simulink model "QD2_DroneStack_PID_2021a"  (R2026a)
settings: Solver=ode1  StopTime=inf  FixedStep=1/1000  EnableMultiTasking=on
InitFcn:
  | Motor_Mapping_7_Inch
model workspace (MAT data in the model file):
  target_system = 1
undefined symbols (not defined in the file): _Commander, _Stabilizer, _SYSID, datetime, HIL, KT, lf, log_, log_QD2_, m, Motor_Matrix, n, qc_get_step_size, s, saved_data
libraries: quarc_library x107, simulink x30, simulink_extras x3, sl_discontinuities x2
(part 5 of 5)

== matlab function QD2_DroneStack_PID_2021a/COMMANDER (ANGLE MODE)/STATE MACHINE TRANSITION ==
  data: current_state input; E_Abort input; isArm input; pt_ARM_to_TAKEOFF_THROTTLE input; pt_TAKE_OFF_HEIGHT_TO_AUTOLAND input; pt_FLIGHT_TO_AUTOLAND input; Next_state output; pt_TAKEOFF_THROTTLE_TO_TAKEOFF_HEIGHT input; pt_TAKE_OFF_HEIGHT_TO_FLIGHT input; pt_AUTOLAND_TO_DISABLE input; pt_EMERGENCY_STOP_TO_DISABLE input; pt_EMERGENCY_ABORT_TO_DISABLE input; Error input
function Next_state = SM_transition(current_state, E_Abort, isArm, pt_ARM_to_TAKEOFF_THROTTLE, pt_TAKE_OFF_HEIGHT_TO_AUTOLAND, pt_FLIGHT_TO_AUTOLAND, pt_TAKEOFF_THROTTLE_TO_TAKEOFF_HEIGHT, pt_TAKE_OFF_HEIGHT_TO_FLIGHT, pt_AUTOLAND_TO_DISABLE, pt_EMERGENCY_STOP_TO_DISABLE, pt_EMERGENCY_ABORT_TO_DISABLE, Error)

% Programmatic Transition Block
%
% FINITE STATE MACHINE (FSM) with 9 states as described below, transitioning based on the 
% values of the isArm, transition signals, Error, and E_Abort
%
% Last modified: March, 2020
%
% INPUTS:
% ------
% current_state = Current state of the FSM        (#)     [1]
% E_Abort                                         (bool)  [1]
% isArm                                           (bool)  [1]
% pt_ARM_TO_TAKEOFF_THROTTLE                      (bool)  [1]
% pt_TAKE_OFF_HEIGHT_TO_AUTOLAND                  (bool)  [1]
% pt_FLIGHT_TO_AUTOLAND                           (bool)  [1]
% pt_TAKEOFF_THROTTLE_TO_TAKEOFF_HEIGHT           (bool)  [1]
% pt_TAKE_OFF_HEIGHT_TO_FLIGHT                    (bool)  [1]
% pt_AUTOLAND_TO_DISABLE                          (bool)  [1]
% pt_EMERGENCY_STOP_TO_DISABLE                    (bool)  [1]
% pt_EMERGENCY_ABORT_TO_DISABLE                   (bool)  [1]
% Error                                           (bool)  [1]
%
% OUTPUT:
% -------
% Next_state = Next state of the FSM              (#)     [1]

Next_state = double(0);
switch current_state
%-------------------------------------------------------------------------%
    case 1 % IDLE STATE
        if E_Abort
            Next_state = 8; % GOTO EMERGENCY ABORT STATE
        elseif Error
            Next_state = 7; % GOTO EMERGENCY STOP STATE
        elseif isArm
            Next_state = 2; % GOTO ARMED STATE
        else
            Next_state = 1; % STAY IN IDLE STATE
        end
%-------------------------------------------------------------------------%
    case 2 % ARMED STATE
        if E_Abort
            Next_state = 8; % GOTO EMERGENCY ABORT STATE
        elseif Error
            Next_state = 7; % GOTO EMERGENCY STOP STATE
        elseif ~isArm
            Next_state = 1; % GOTO IDLE STATE
        elseif pt_ARM_to_TAKEOFF_THROTTLE
            Next_state = 3; % GOTO TAKEOFF_THROTTLE STATE 
        else
            Next_state = 2; % STAY IN ARMED STATE
        end
%-------------------------------------------------------------------------%
    case 3 % TAKEOFF_THROTTLE STATE
        if E_Abort
            Next_state = 8; % GOTO EMERGENCY ABORT STATE
        elseif Error
            Next_state = 7; % GOTO EMERGENCY STOP STATE
        elseif pt_TAKEOFF_THROTTLE_TO_TAKEOFF_HEIGHT
            Next_state = 4; % GOTO TAKEOFF_HEIGHT STATE
        else
            Next_state = 3; % STAY IN TAKEOFF_THROTTLE STATE
        end
%-------------------------------------------------------------------------%
    case 4 % TAKEOFF_HEIGHT STATE
        if E_Abort
            Next_state = 8; % GOTO EMERGENCY ABORT STATE
        elseif Error
            Next_state = 7; % GOTO EMERGENCY STOP STATE
        elseif pt_TAKE_OFF_HEIGHT_TO_AUTOLAND
            Next_state = 6;
        elseif pt_TAKE_OFF_HEIGHT_TO_FLIGHT
            Next_state = 5; % GOTO FLIGHT STATE
        else
            Next_state = 4; % STAY IN TAKEOFF_HEIGHT STATE
        end
%-------------------------------------------------------------------------%
    case 5 % FLIGHT STATE
        if E_Abort
            Next_state = 8; % GOTO EMERGENCY ABORT STATE
        elseif Error
            Next_state = 7; % GOTO EMERGENCY STOP STATE
        elseif pt_FLIGHT_TO_AUTOLAND
            Next_state = 6; % GOTO AUTO_LAND STATE
        else
            Next_state = 5; % STAY IN FLIGHT STATE
        end
%-------------------------------------------------------------------------%       
    case 6 % AUTO_LAND STATE
        if E_Abort
            Next_state = 8; % GOTO EMERGENCY ABORT STATE
        elseif Error
            Next_state = 7; % GOTO EMERGENCY STOP STATE
        elseif pt_AUTOLAND_TO_DISABLE
            Next_state = 9; % GOTO DISABLE STATE
        else
            Next_state = 6; % STAY IN AUTO_LAND STATE
        end
%-------------------------------------------------------------------------%
    case 7 % EMERGENCY STOP STATE
        if E_Abort
            Next_state = 8; % GOTO EMERGENCY ABORT STATE
        elseif pt_EMERGENCY_STOP_TO_DISABLE
            Next_state = 9; % GOTO DISABLE STATE
        else
            Next_state = 7; % STAY IN EMERGENCY STOP STATE
        end
%-------------------------------------------------------------------------%
    case 8 % EMERGENCY ABORT
        if pt_EMERGENCY_ABORT_TO_DISABLE
            Next_state = 9; % GOTO DISABLE STATE
        else 
            Next_state = 8; % STAY IN EMERGENCY ABORT STATE
        end
%-------------------------------------------------------------------------%    
    case 9 % DISABLE
        Next_state = 9; % Always stay in DISABLE state if you are here    
end

== matlab function QD2_DroneStack_PID_2021a/Communication/Detect Communication Loss/MATLAB Function ==
  settings: updateMethod=DISCRETE
  data: time input; stream_connection_loss output; state input; error input; ms_time input; data_loss output
function [stream_connection_loss , data_loss] = fcn(time, state, error, ms_time)

persistent ms_time_prev
    if isempty(ms_time_prev)
        ms_time_prev = 0;
    end

stream_connection_loss = 0;
data_loss = 0;
if time > 3
    if ((state ~= 2)&&(error < 0))
        % stream connection is not established correctly
        stream_connection_loss = 1;
    end

    if (ms_time == ms_time_prev)&&(ms_time > 0)
        % data is stale
        data_loss = 1;
    end
end

ms_time_prev = ms_time;

== matlab function QD2_DroneStack_PID_2021a/QDrone 2 DAQ/Attitude Estimate from IMU Data/For Each Subsystem - Iterate over IMU0 and IMU1/Roll and Pitch Approximation from Accelerometer data ==
  data: acc_body input; roll_acc output; pitch_acc output
function [roll_acc, pitch_acc]   = fcn(acc_body)
%#eml
n = norm(acc_body,2);
if n>eps
    acc_body = acc_body/n; 
else
    acc_body = [0 0 1]';
end

roll_acc = atan2(acc_body(2),acc_body(3));
pitch_acc = atan2( -acc_body(1), acc_body(2)*sin(roll_acc)+acc_body(3)*cos(roll_acc));

== matlab function QD2_DroneStack_PID_2021a/QDrone 2 DAQ/Choose Motor Telemetry/MATLAB Function ==
  data: enable input; idx output; n input
function idx = num_seq(enable, n)

% Generate a running sequence of number from 0 to n
persistent state 

if isempty(state)
    state = 0;
end

% Output state index
idx = state;

if enable
    % Increment state index
    state = state + 1;
    % Check state index, reset when needed
    if state >= n
        state = 0;
    end
else
    % reset state to zero and not requesting telemetry
    state = 0;
    idx = 0;
end

== matlab function QD2_DroneStack_PID_2021a/QDrone 2 DAQ/Detect ESC Problems/MATLAB Function ==
  settings: updateMethod=DISCRETE  sampleTime=qc_get_step_size
  data: u input; n output; buffer_size input
function n = count_pulses(u, buffer_size)

persistent idx
persistent buffer

if( isempty(idx) )
    idx = 1;
end
if( isempty(buffer) )
    buffer = zeros(length(u),buffer_size);
end

% Initialize output vector
n = zeros(length(u),1);

% Store value into buffer
buffer(:,idx) = u;
% Increment index value
idx = idx + 1;
if idx > buffer_size
    % Reset index counter
    idx = 1;
end

% Add up all pulses (1) along each row in the buffer
n = sum(buffer,2);

== matlab function QD2_DroneStack_PID_2021a/QDrone 2 DAQ/MATLAB Function ==
  data: mdl_time input; arm input; estop input; esc_problem input; cmd output; cmd_enable output; tele_enable output; esc_ready output; esc_timeout output; stop_mdl output; pre_state input; state output
function [cmd, cmd_enable, tele_enable, esc_ready, esc_timeout, stop_mdl, state] = esc_state_machine(mdl_time, arm, estop, esc_problem, pre_state)

persistent next_state_after_pause
persistent state_counter
persistent state_counter_after_pause
persistent esc_timeout_state

% Define state enumeration
STATE_INIT_WAIT = 0;
STATE_INIT_WAIT_EXTENDED = 1;
STATE_IDLE = 2;
STATE_CMD_BEEP = 3;
STATE_CMD_SET_DIRECTION = 4;
STATE_CMD_MOTOR = 5;
STATE_CMD_ZERO = 77;
STATE_CMD_DISABLED = 88;
STATE_EXIT = 99;

% Define state counter values
COUNT_STATE_INIT_MIN = 1000;
COUNT_STATE_INIT_MAX = 10000;
COUNT_STATE_IDLE = 1000;
COUNT_STATE_BEEP = 60;
%COUNT_STATE_BEEP = 1000;
COUNT_STATE_SET_DIRECTION = 120;
%COUNT_STATE_SET_DIRECTION = 500;
COUNT_STATE_DISABLE_BEEP = 1000;
COUNT_STATE_DISABLE_DIRECTION = 500;
COUNT_STATE_CMD_ZERO_PAUSE = 1000;


% Initialize persistent variables
if isempty(next_state_after_pause)
    next_state_after_pause = STATE_EXIT;
end
if isempty(state_counter)
    state_counter=COUNT_STATE_INIT_MIN;
end
if isempty(state_counter_after_pause)
    state_counter_after_pause = COUNT_STATE_IDLE;
end
if isempty(esc_timeout_state)
    esc_timeout_state = 0;
end


% Initialize output
state = STATE_INIT_WAIT;
cmd = [0,0,0,0];
tele_enable = 0;
cmd_enable = 0;
stop_mdl = 0;
esc_ready = 0;

% State Transition
% E-Stop superceeds all commands
if estop
    state = STATE_EXIT;
else
    switch pre_state
        % Initialization - send command zero and request telemetry
        case STATE_INIT_WAIT
            state_counter = state_counter - 1;
            if state_counter <= 0 
                % Go to next state
                state = STATE_INIT_WAIT_EXTENDED;
                state_counter = COUNT_STATE_INIT_MAX;
            else
                % Stay in current state
                state = pre_state;
            end
    
    
        % Extended initialization wait until ESC initialization completed
        case STATE_INIT_WAIT_EXTENDED
            state_counter = state_counter - 1;
            if state_counter <= 0
                % Max timeout reached, unrecoverable error condition, flag and
                % terminate.
                state = STATE_EXIT;
                esc_timeout_state = 1;
                
            else
                % Check if we are clear to proceed
                if esc_problem
                    % Stay in current state and keep waiting
                    state = pre_state;
                else
                    % Go to next state
                    state = STATE_CMD_ZERO;
                    state_counter = COUNT_STATE_CMD_ZERO_PAUSE;
                    next_state_after_pause = STATE_CMD_BEEP;
                    state_counter_after_pause = COUNT_STATE_BEEP;
                end
            end
    
        % Send Beep command
        case STATE_CMD_BEEP
            state_counter = state_counter - 1;
            if state_counter <= 0
                % Go to next state
                state = STATE_CMD_DISABLED;
                state_counter = COUNT_STATE_DISABLE_BEEP;
                next_state_after_pause = STATE_CMD_SET_DIRECTION;
                state_counter_after_pause = COUNT_STATE_SET_DIRECTION;
                % Alternately go directly to set direction
%                 state = STATE_CMD_SET_DIRECTION;
%                 state_counter = COUNT_STATE_SET_DIRECTION;
            else
                % Stay in current state
                state = pre_state;
            end
            
        % Set Direction
        case STATE_CMD_SET_DIRECTION
            state_counter = state_counter - 1;
            if state_counter <= 0
                % Go to next state
                state = STATE_CMD_DISABLED;
                state_counter = COUNT_STATE_DISABLE_DIRECTION;
                next_state_after_pause = STATE_IDLE;
                state_counter_after_pause = COUNT_STATE_IDLE;
            else
                % Stay in current state
                state = pre_state;
            end
    
        % Idle/Disarm state with telemetry enabled
        case STATE_IDLE
            if arm
                % Go to next state
                state = STATE_CMD_MOTOR;
            else
                % Stay and wait
                state = pre_state;
            end
            
        % Drive motor
        case STATE_CMD_MOTOR
            % Skip checking for telemetry fails after motor starts
%            if not(esc_problem)
                if not(arm)
                    % Go to next state
                    state = STATE_IDLE;
                else
                    % Stay in current state
                    state = pre_state;
                end
%             else
%                 % Not expecting this but flag it
%                 state = STATE_EXIT;
%                 esc_timeout_state = 1;
%             end
    
        % Pause with command disabled
        case STATE_CMD_DISABLED
            state_counter = state_counter - 1;
            if state_counter <= 0
                % Go to next state
                state = next_state_after_pause;
                state_counter = state_counter_after_pause;
            else
                % stay in current state
                state = pre_state;
            end
            
        % Generic pause state with command and telemetry enabled
        case STATE_CMD_ZERO
            state_counter = state_counter - 1;
            if state_counter <= 0
                % Got to next state
                state = next_state_after_pause;
                state_counter = state_counter_after_pause;
            else
                % Stay in current state
                state = pre_state;
            end 

        % Exit state
        case STATE_EXIT
            % Do nothing until model stop
            state = pre_state;
    end
end

% State Output
switch state
    % Command zero to initialize the ESC
    case STATE_INIT_WAIT
        cmd = [0, 0, 0, 0];
        tele_enable = 1;
        cmd_enable = 1;
        stop_mdl = 0;
        esc_ready = 0;

    % Extended wait during initialization to confirm all ESC are ready
    case STATE_INIT_WAIT_EXTENDED
        cmd = [0,0,0,0];
        tele_enable = 1;
        cmd_enable = 1;
        stop_mdl = 0;
        esc_ready = 0;

    % Send beep command
    case STATE_CMD_BEEP
        cmd = [1, 1, 1, 1]*3;
        %tele_enable = 0;
        % Old BLHeli firmware needs the telemetry bit set to accept beep
        % command
        tele_enable = 1;
        cmd_enable = 1;
        stop_mdl = 0;
        esc_ready = 0;

    % Set Direction
    case STATE_CMD_SET_DIRECTION
        % Normal - for old BLHeli firmware
        cmd = [20, 21, 21, 20];
        % Workaround - for new AM32 firmware - looks like a bug  
        %cmd = [21, 20, 20, 21];
        %cmd = [21, 21, 21, 21];
        %cmd = [20, 20, 20, 20];
        %tele_enable = 0;
        % old BLHeli firmware needs the telemetry bit set to accept set
        % direction command
        tele_enable = 1;
        cmd_enable = 1;
        stop_mdl = 0;
        esc_ready = 0;

    % Disarm command
    case STATE_IDLE
        cmd = [0,0,0,0];
        tele_enable = 0;
        cmd_enable = 1;
        stop_mdl = 0;
        esc_ready = 1;
        
    % Drive motors
    case STATE_CMD_MOTOR
        cmd = [48, 48, 48, 48];
        tele_enable = 1;
        cmd_enable = 1;
        stop_mdl = 0;
        esc_ready = 1;

    % Idle/disable state
    case STATE_CMD_DISABLED
        cmd = [0 0 0 0];
        tele_enable = 0;
        cmd_enable = 0;
        stop_mdl = 0;
        esc_ready = 0;

    % Generic Pause
    case STATE_CMD_ZERO
        cmd = [0,0,0,0];
        tele_enable = 1;
        cmd_enable = 1;
        stop_mdl = 0;
        esc_ready = 0;

    % Stop
    case STATE_EXIT
        cmd = [0,0,0,0];
        tele_enable = 0;
        cmd_enable = 1;
        stop_mdl = 1;
        esc_ready = 0;
end

% output esc_timeout variable
esc_timeout = esc_timeout_state;

== matlab function QD2_DroneStack_PID_2021a/QDrone 2 DAQ/Force to percentage Mapping ==
  data: V_Bat_Act input; Motor_Forces input; Duty_Cycle output; KT input
function Duty_Cycle = fcn(V_Bat_Act,Motor_Forces,KT)

B = KT(2)^2-4*KT(1)*(KT(3)-Motor_Forces)

invalid_signal = B < 0
B(invalid_signal) = 0

% Ranges from 1000-2000
Volt_CMD_Theo = -0.5*KT(2)/KT(1)+ sqrt(B)/(2*KT(1));

Duty_Cycle = Volt_CMD_Theo/V_Bat_Act;

== matlab function QD2_DroneStack_PID_2021a/STABILIZER - QDRONE 2/SYSID Axis Router ==
  data: u input; axis input; momentSweep output; thrustSweep output
function [momentSweep,thrustSweep] = routeSweep(u,axis)
%#codegen

momentSweep = [0.0 0.0 0.0];
thrustSweep = 0.0;

if axis == 1
    momentSweep(1) = u;      % roll moment
elseif axis == 2
    momentSweep(2) = u;      % pitch moment
elseif axis == 3
    momentSweep(3) = u;      % yaw moment
elseif axis == 4
    thrustSweep = u;         % collective thrust
end

== matlab function QD2_DroneStack_PID_2021a/COMMANDER (ANGLE MODE)/THROTTLE SWITCHBOX /Throttle Switchbox ==
  data: FSM_state input; sigmoid output
function sigmoid  = application_drone_throttle_switchbox(FSM_state)

% Application Drone: Throttle Switchbox
%
% Logic for switching between throttle commands from the controller 
%
% v2.0 - 5th october, 2018
%
% INPUTS:
% -------
% FSM_state = current state of the FSM------------------------------------------------------- (#)         [1]
% 
% OUTPUTS:
% --------
% sigmoid = an integer whose state determines how the heights are transformed---------------- (#)         [1]
% sigmoid = 1 - Command 0 throttle
% sigmoid = 2 - Sigmoid throttle up from 0 to the trim value
% sigmoid = 3 - Pass controller throttle straight through + trim value.
% sigmoid = 4 - Ignore controller throttle. Sigmoid it down to 0.
% sigmoid = 5 - Pass controller throttle straight through + trim value.


sigmoid = 0;
switch FSM_state
    case 1 % IDLE STATE
        sigmoid = 1;
    case 2 % ARM STATE
        sigmoid = 1;
    case 3 % TAKEOFF THROTTLE STATE
        sigmoid = 2;
    case 4 % TAKEOFF HEIGHT STATE
        sigmoid = 3;
    case 5 % FLIGHT STATE
        sigmoid = 3;
    case 6 % AUTOLAND STATE
        sigmoid = 5;
    case 7 % EMERGENCY STOP STATE
        sigmoid = 4;
    case 8 % EMERGENCY ABORT STATE
        sigmoid = 1;
    case 9 % DISABLE STATE
        sigmoid = 1;
end

== matlab function QD2_DroneStack_PID_2021a/STABILIZER - QDRONE 2/MATLAB Function ==
  settings: updateMethod=DISCRETE
  data: u output; request input; A input; w0 input; w1 input; T input; tramp input; active output; omega output; t input; safe input
function [u,active,omega] = logSweep( ...
    request,A,w0,w1,T,tramp,t,safe)
%#codegen

persistent tStart previousRequest aborted

if isempty(tStart)
    tStart = 0.0;
    previousRequest = false;
    aborted = false;
end

u = 0.0;
active = 0.0;
omega = 0.0;

enabled = request > 0.5;
safeNow = safe > 0.5;

% Turning the request off rearms the generator.
if ~enabled
    previousRequest = false;
    aborted = false;
    return
end

% Any unsafe condition aborts the maneuver.
if ~safeNow
    previousRequest = true;
    aborted = true;
    return
end

% Start only on a new request.
if ~previousRequest
    tStart = t;
end

previousRequest = true;

% An aborted maneuver cannot resume until request is toggled off.
if aborted
    return
end

tau = t - tStart;

valid = tau >= 0.0 && tau <= T && ...
    T > 0.0 && w0 > 0.0 && w1 > 0.0;

if valid
    beta = log(w1/w0)/T;

    if abs(beta) < 1.0e-9
        omega = w0;
        phase = w0*tau;
    else
        exponentialTerm = exp(beta*tau);
        omega = w0*exponentialTerm;
        phase = (w0/beta)*(exponentialTerm - 1.0);
    end

    ramp = max(0.0,min(tramp,T/2.0));
    envelope = 1.0;

    if ramp > 0.0
        if tau < ramp
            envelope = 0.5*(1.0-cos(pi*tau/ramp));
        elseif tau > T-ramp
            envelope = 0.5*(1.0-cos(pi*(T-tau)/ramp));
        end
    end

    u = A*envelope*sin(phase);
    active = 1.0;
end

== matlab function QD2_DroneStack_PID_2021a/HORIZON FRAME CONVERSION AND ESTIMATION/Pose Switchbox/MATLAB Function ==
  data: sigmoid_type input; enable output; x_des input; slow_lim input; fast_lim input; x_cur input; x_vel input; x_ref output; max_x_vel output; max_x_accel output; x_meas input
function [enable, x_ref, max_x_vel, max_x_accel] = fcn(sigmoid_type, x_des, slow_lim, fast_lim, x_cur, x_vel, x_meas)

% Note: Some of the cases below are identical. However, they are separated out 
% based on the states of the state machine for ease of modification in the future. 
% For example, states 4 and 5 are identical. However, if the user wants different 
% signmoid behaviour when taking off than when landing, these cases may not be the same. 

enable = 0;
x_ref = 0;
max_x_vel = 0;
max_x_accel = 0;

switch sigmoid_type
    case 1 % This is for the IDLE, ARM, E_ABORT, E_STOP and DISABLE states of the FSM
        enable = 1;
        x_ref = x_meas;
        max_x_vel = slow_lim(1);
        max_x_accel = slow_lim(2);

    case 2 % This is for the TAKEOFF THROTTLE state of the FSM
        enable = 1;
        x_ref = x_meas;
        max_x_vel = slow_lim(1);
        max_x_accel = slow_lim(2);

    case 3 % This is for the FLIGHT state of the FSM
        enable = 1;
        x_ref = x_des;
        max_x_vel = fast_lim(1);
        max_x_accel = fast_lim(2);

    case 4 % This is for the TAKEOFF HEIGHT state of the FSM
        enable = 1;
        x_ref = x_des;
        if (abs(x_cur - x_des) <= 0.02)
            max_x_vel = fast_lim(1);
            max_x_accel = fast_lim(2);
        else    
            max_x_vel = slow_lim(1);
            max_x_accel = slow_lim(2);
        end
    case 5 % This is for the AUTOLAND state of the FSM
        enable = 1;
        x_ref = x_des;
        if (abs(x_cur - x_des) <= 0.02)
            max_x_vel = fast_lim(1);
            max_x_accel = fast_lim(2);        
        else
            max_x_vel = slow_lim(1);
            max_x_accel = slow_lim(2);
        end
        
end

== matlab function QD2_DroneStack_PID_2021a/HORIZON FRAME CONVERSION AND ESTIMATION/Pose Switchbox/MATLAB Function1 ==
  data: sigmoid_type input; enable output; y_des input; slow_lim input; fast_lim input; y_cur input; y_vel input; y_ref output; max_y_vel output; max_y_accel output; y_meas input
function [enable, y_ref, max_y_vel, max_y_accel] = fcn(sigmoid_type, y_des, slow_lim, fast_lim, y_cur, y_vel, y_meas)

% Note: Some of the cases below are identical. However, they are separated out 
% based on the states of the state machine for ease of modification in the future. 
% For example, states 4 and 5 are identical. However, if the user wants different 
% signmoid behaviour when taking off than when landing, these cases may not be the same. 

enable = 0;
y_ref = 0;
max_y_vel = 0;
max_y_accel = 0;

switch sigmoid_type
    case 1 % This is for the IDLE, ARM, E_ABORT, E_STOP and DISABLE states of the FSM
        enable = 1;
        y_ref = y_meas;
        max_y_vel = slow_lim(1);
        max_y_accel = slow_lim(2);

    case 2 % This is for the TAKEOFF THROTTLE state of the FSM
        enable = 1;
        y_ref = y_meas;
        max_y_vel = slow_lim(1);
        max_y_accel = slow_lim(2);

    case 3 % This is for the FLIGHT state of the FSM
        enable = 1;
        y_ref = y_des;
        max_y_vel = fast_lim(1);
        max_y_accel = fast_lim(2);

    case 4 % This is for the TAKEOFF HEIGHT state of the FSM
        enable = 1;
        y_ref = y_des;
        if (abs(y_cur - y_des) <= 0.02)
            max_y_vel = fast_lim(1);
            max_y_accel = fast_lim(2);
        else    
            max_y_vel = slow_lim(1);
            max_y_accel = slow_lim(2);
        end
    case 5 % This is for the AUTOLAND state of the FSM
        enable = 1;
        y_ref = y_des;
        if (abs(y_cur - y_des) <= 0.02)
            max_y_vel = fast_lim(1);
            max_y_accel = fast_lim(2);        
        else
            max_y_vel = slow_lim(1);
            max_y_accel = slow_lim(2);
        end
        
end
